simulink model "stepchange_timevarying_change"  (R2022b)
settings: Solver=VariableStepAuto  StartTime=0.0  StopTime=8  RelTol=1e-3
values from neighbouring files (symbols this model uses):
  A = [eye(N),     -LoadZ^-1,   B; zeros(BN,N),  R_l^-1*B',   eye(BN); zeros(1,N),  zeros(1,N),   V_r'*B ]    [stepchange_timevarying_change_initial_document.m]
  A_r = kron(diag(r),eye(N+BN+1))    [stepchange_timevarying_change_initial_document.m]
  alpha_u = [1.1    1.4    1.8    1.1           1.1    1.9    1.9    1.2           1.3    1.4    1.8    0.6           1.8    2.1    1.5    0.9]'    [stepchange_timevarying_change_initial_document.m]
  alpha_V = [0.7    0.6    0.8    0.9           0.7    1.2    0.8    1.24           0.3    0.3    0.0    1.70           1.0    0.5    1.1    1.0]'    [stepchange_timevarying_change_initial_document.m]
  alpha_w = 0.8    [stepchange_timevarying_change_initial_document.m]
  BN = size(Line1,1)/2    [stepchange_timevarying_change_initial_document.m]
  bound_up_vector = zeros(3*N,1)    [stepchange_timevarying_change_initial_document.m]
  changerate = 3    [stepchange_timevarying_change_initial_document.m]
  changetime = 5    [stepchange_timevarying_change_initial_document.m]
  changevariance = 0.1    [stepchange_timevarying_change_initial_document.m]
  constraint_gain = 200    [stepchange_timevarying_change_initial_document.m]
  Dw = 0.01    [stepchange_timevarying_change_initial_document.m]
  epsilon = 2    [stepchange_timevarying_change_initial_document.m]
  F_x = blkdiag(diag(r)*diag(alpha_I)+diag(r)*pr*diag(V_r),diag(r)*diag(alpha_V),F_x_I)    [stepchange_timevarying_change_initial_document.m]
  kappa = 10    [stepchange_timevarying_change_initial_document.m]
  l = 2.5    [stepchange_timevarying_change_initial_document.m]
  lambda_ini = zeros(N*(BN+N+1),1)    [stepchange_timevarying_change_initial_document.m]
  Lap = 1000*(Degree-Adjacent)    [stepchange_timevarying_change_initial_document.m]
  Lap_BN_plus_N = kron(Lap,eye(BN+N+1))    [stepchange_timevarying_change_initial_document.m]
  Lineconstrants = 10*ones(BN,1)    [stepchange_timevarying_change_initial_document.m]
  Lineindex = zeros(BN,4)    [stepchange_timevarying_change_initial_document.m]
  LoadI = [30.0;15.0;30.0;26.0;         18.9;22.8;29.6;32.1;         22.6;27.6;16.5;19.9;         26.5;19.4;22.7;24.9]    [stepchange_timevarying_change_initial_document.m]
  LoadIchange = [30.0;15.0;30.0;26.0;         18.9;22.8;29.6;32.1;         22.6;27.6;16.5;19.9;         26.5;19.4;22.7;24.9]+3*ones(N,1)    [stepchange_timevarying_change_initial_document.m]
  LoadIchangeno = 3    [stepchange_timevarying_change_initial_document.m]
  LoadZ = diag([16.7;50.0;16.7;20.0;              25.0;16.0;14.2;29.4;              18.5;19.6;22.6;25.6;              23.4;26.4;25.2;33.7])    [stepchange_timevarying_change_initial_document.m]
  LoadZchange = diag([16.7;50.0;16.7;20.0;              25.0;16.0;14.2;29.4;              18.5;19.6;22.6;25.6;              23.4;26.4;25.2;33.7])+3*diag(ones(N,1))    [stepchange_timevarying_change_initial_document.m]
  LoadZchangeno = 3    [stepchange_timevarying_change_initial_document.m]
  N = 16    [stepchange_timevarying_change_initial_document.m]
  NCLN = zeros(N,1)    [stepchange_timevarying_change_initial_document.m]
  normal_vector = zeros(3*N,1)    [stepchange_timevarying_change_initial_document.m]
  nu_ini = [-0.00758212493845042	-0.0182492317603708	0.00714905390846842	0.0186908981861182          -0.00758212493845042	-0.0182492317603708	0.00714905390846842	0.0186908981861182          -0.00758212493845042	-0.0182492317603708	0.00714905390846842	0.0186908981861182          -0.00758212493845042	-0.0182492317603708	0.00714905390846842	0.0186908981861182]'    [stepchange_timevarying_change_initial_document.m]
  pr = 0.005    [stepchange_timevarying_change_initial_document.m]
  r = [1.06 1.03 1.05 1.04     1.02 1.03 1.04 1.01     1.03 1.04 1.06 1.07     1.01 1.03 1.04 1.02]    [stepchange_timevarying_change_initial_document.m]
  s_A = zeros(N*(N+BN+1),1)    [stepchange_timevarying_change_initial_document.m]
  theta_ini = zeros(N*(BN+N+1),1)    [stepchange_timevarying_change_initial_document.m]
  u_ini = [378.9289  380.4146  379.7396  379.2243  380.1955  381.1042         379.9247  379.8974  380.0252  380.4045  379.6763  379.8341         380.1194  380.5682  379.3881  379.9696]'    [stepchange_timevarying_change_initial_document.m]
  upsilon_ini = [172.552238898892	172.552238898892	172.552238898892	172.552238898892               172.552238898892	172.552238898892	172.552238898892	172.552238898892               172.552238898892	172.552238898892	172.552238898892	172.552238898892               172.552238898892	172.552238898892	172.552238898892	172.552238898892]'    [stepchange_timevarying_change_initial_document.m]
  V_hat_low = (380-3)*ones(N,1)    [stepchange_timevarying_change_initial_document.m]
  V_hat_up = (380+3)*ones(N,1)    [stepchange_timevarying_change_initial_document.m]
  V_r = [380.16  381.31  380.27  380.13       380.12  381.24  380.15  380.35       380.15  381.13  380.09  380.22       380.19  381.26  380.21  380.19]'    [stepchange_timevarying_change_initial_document.m]
  varepsilon = 50    [stepchange_timevarying_change_initial_document.m]
  x_hat_ini = [14.515064754915	3.95935897697232	32.9787419273847	14.9071228299889             37.6257931691129	61.1095883901259	41.4721611959256	33.6364102939300             44.9867290171943	52.8132621486412	28.1355733315040	33.0707668633162             36.6024320622732	49.3936276267038	2.38033527987224	36.4476162672594             378.638597580330	380.343321138855	379.211948658584	379.000752058610              ...(+639 chars)    [stepchange_timevarying_change_initial_document.m]
undefined symbols (not defined in the file or in its folder): bound_low_vector
libraries: fl_lib x204, nesl_utility x101, simulink x2, spspowerguiLib x1
(part 1 of 3)
settings Model: Creator=27843  LastModifiedBy=27843

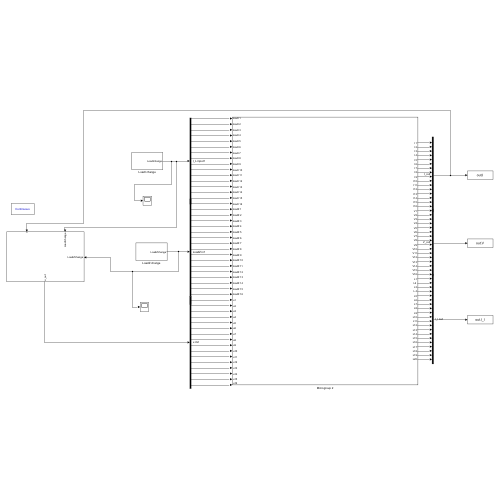
[thumbnail: Simulink's stored preview of the top-level diagram]
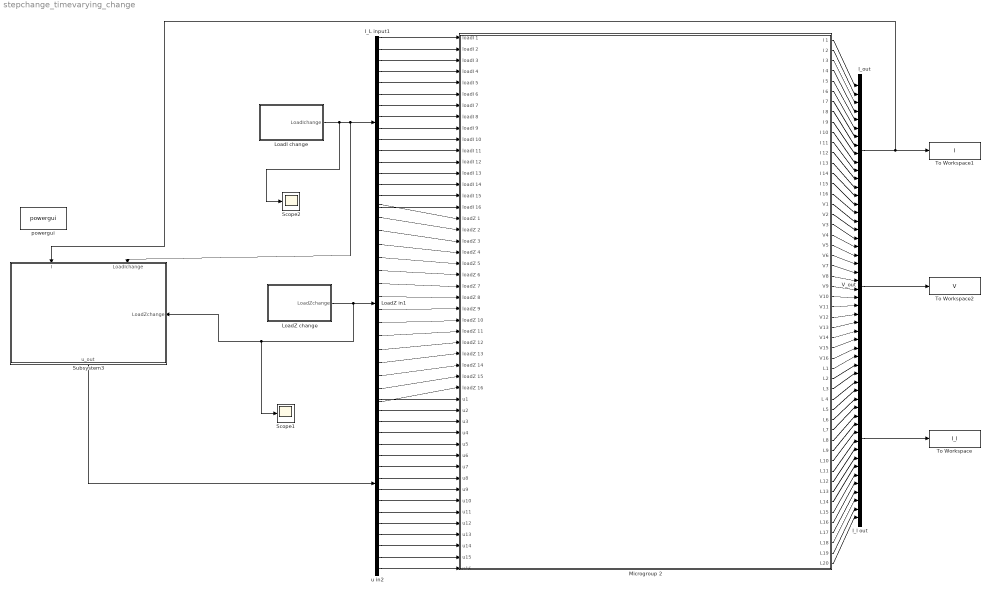
== system stepchange_timevarying_change ==
  I_L input1 : Demux  Outputs=16
  I_l out : Mux  Inputs=20
  I_out : Mux  Inputs=16
  LoadI change : Subsystem
  LoadZ change : Subsystem
  LoadZ in1 : Demux  Outputs=16
  Microgroup 2 : Subsystem
  Scope1 : Scope
  Scope2 : Scope
  Subsystem3 : Subsystem
      settings: PortSchema="{\"entries\":[{\"content\":{\"sides\":[{\"content\":{\"connectorIds\":[\"In1\",\"In2\"]},\"type\":\"ConnectorPlacement.EquallySpacedRectSide\",\"uuid\":\"fae7fbbb-70cd-4db5-acb5-97da1dd1ec52\"},{\"content\":{\"connectorIds\":[\"Out1\"],\"side\":\"RIGHT\"},\"type\":\"ConnectorPlacement.EquallySpacedRectSide\",\"uuid\":\"fa6dcfc8-22a3-4b8e-9bd6-bb4867dcf5b7\"},{\"content\":{\"connectorIds\":[],\"side\":\"TOP\"},\"type\":\"ConnectorPlacement.EquallySpacedRectSide\",\"uuid\":\"9780a6fc-e699-499b-ab3e-b386f79a2eae\"},{\"content\":{\"connectorIds\":[\"In3\"],\"side\":\"BOTTOM\"},\"type\":\"ConnectorPlacement.EquallySpacedRectSide\",\"uuid\":\"c19162d8-377f-47b4-a15d-68590b7e29f2\"}]},\"type\":\"ConnectorPlacement.EquallySpacedConnector\",\"uuid\":\"94524866-4569-4101-9a5a-19d024da94d3\"}],\"packageUris\":[\"http://schema.mathworks.com/mf0/Connector/R2020b\"],\"version\":\"1.0\"}"
  To Workspace : ToWorkspace  VariableName=I_l  SaveFormat=Timeseries  SampleTime=-1
  To Workspace1 : ToWorkspace  VariableName=I  SaveFormat=Timeseries  SampleTime=-1
  To Workspace2 : ToWorkspace  VariableName=V  SaveFormat=Timeseries  SampleTime=-1
  V_out : Mux  Inputs=16
  powergui : spspowerguiLib/powergui  Priority=1  SimulationMode=Continuous  SampleTime=50e-6  frequency=60  Iterations=50  frequencyindice=60  Pbase=100e6  ErrMax=1e-4  UnitsV=kV  UnitsW=MW  buscounter=0  FunctionMessages=off  echomessages=off  EnableUseOfTLC=off  CurrentSourceSwitches=off  DisableSnubberDevices=off  DisableRonSwitches=off  DisableVfSwitches=off  DisplayEquations=off  AutomaticDiscreteSolvers=off  SolverType=Tustin/Backward Euler (TBE)  Interpol=off  ExternalGateDelay=off  methode=off  Ts=100  x0status=blocks  SPID=on  SwTol=0  HookPort=off  NonlinearTolerance=1e-4  nMaxIteration=100  ContinueOnMaxIteration=off  RestoreLinks=warning  ResistiveCurrentMeasurement=off  Frange=[0:2:500]  Ylog=off  Xlog=on  ShowGrid=off  save=off  variable=ZData  structure=0  ZoomFFT=off  StartTime=0.0  cycles=1  DisplayStyle=1  fundamental=60  FreqAxis=off  MaxFrequency=1000  frequencyindicesteady=1  RmsSteady=1  display=off
  u in2 : Demux  Outputs=16
  wires:
  Microgroup 2/25(V9) -> V_out/9
  Microgroup 2/11(I 11) -> I_out/11
  I_L input1/14 -> Microgroup 2/14(loadI 14)
  LoadI change/1(LoadIchange) -> Scope2/1, I_L input1/1, Subsystem3/2(LoadIchange)
  Microgroup 2/23(V7) -> V_out/7
  LoadZ change/1(LoadZchange) -> Scope1/1, Subsystem3/3(LoadZchange), LoadZ in1/1
  Microgroup 2/20(V4) -> V_out/4
  V_out/1 -> To Workspace2/1
  Microgroup 2/8(I 8) -> I_out/8
  Microgroup 2/27(V11) -> V_out/11
  LoadZ in1/3 -> Microgroup 2/19(loadZ 3)
  I_L input1/10 -> Microgroup 2/10(loadI 10)
  u in2/13 -> Microgroup 2/45(u13)
  LoadZ in1/10 -> Microgroup 2/26(loadZ 10)
  u in2/11 -> Microgroup 2/43(u11)
  I_L input1/5 -> Microgroup 2/5(loadI 5)
  I_L input1/8 -> Microgroup 2/8(loadI 8)
  Subsystem3/1(u_out) -> u in2/1
  I_L input1/16 -> Microgroup 2/16(loadI 16)
  u in2/15 -> Microgroup 2/47(u15)
  LoadZ in1/11 -> Microgroup 2/27(loadZ 11)
  I_l out/1 -> To Workspace/1
  LoadZ in1/9 -> Microgroup 2/25(loadZ 9)
  I_out/1 -> To Workspace1/1, Subsystem3/1(I)
  u in2/12 -> Microgroup 2/44(u12)
  Microgroup 2/15(I 15) -> I_out/15
  LoadZ in1/5 -> Microgroup 2/21(loadZ 5)
  u in2/4 -> Microgroup 2/36(u4)
  Microgroup 2/6(I 6) -> I_out/6
  u in2/5 -> Microgroup 2/37(u5)
  u in2/7 -> Microgroup 2/39(u7)
  u in2/8 -> Microgroup 2/40(u8)
  u in2/2 -> Microgroup 2/34(u2)
  LoadZ in1/6 -> Microgroup 2/22(loadZ 6)
  Microgroup 2/51(L19) -> I_l out/19
  I_L input1/3 -> Microgroup 2/3(loadI 3)
  Microgroup 2/39(" L7") -> I_l out/7
  u in2/3 -> Microgroup 2/35(u3)
  u in2/1 -> Microgroup 2/33(u1)
  LoadZ in1/4 -> Microgroup 2/20(loadZ 4)
  Microgroup 2/48(L16) -> I_l out/16
  Microgroup 2/42(L10) -> I_l out/10
  Microgroup 2/41(L9) -> I_l out/9
  Microgroup 2/46(L14) -> I_l out/14
  Microgroup 2/36(L 4) -> I_l out/4
  Microgroup 2/44(L12) -> I_l out/12
  Microgroup 2/38(L6) -> I_l out/6
  Microgroup 2/16(I 16) -> I_out/16
  Microgroup 2/47(L15) -> I_l out/15
  Microgroup 2/14(I 14) -> I_out/14
  Microgroup 2/13(I 13) -> I_out/13
  u in2/10 -> Microgroup 2/42(u10)
  Microgroup 2/22(V6) -> V_out/6
  Microgroup 2/49(L17) -> I_l out/17
  Microgroup 2/33(L1) -> I_l out/1
  Microgroup 2/52(L20) -> I_l out/20
  u in2/14 -> Microgroup 2/46(u14)
  Microgroup 2/18(V2) -> V_out/2
  Microgroup 2/26(V10) -> V_out/10
  u in2/6 -> Microgroup 2/38(u6)
  Microgroup 2/17(V1) -> V_out/1
  Microgroup 2/21(V5) -> V_out/5
  Microgroup 2/50(L18) -> I_l out/18
  Microgroup 2/29(V13) -> V_out/13
  Microgroup 2/19(V3) -> V_out/3
  Microgroup 2/2(I 2) -> I_out/2
  Microgroup 2/43(" L11") -> I_l out/11
  Microgroup 2/7(I 7) -> I_out/7
  LoadZ in1/1 -> Microgroup 2/17(loadZ 1)
  Microgroup 2/5(I 5) -> I_out/5
  Microgroup 2/40(L8) -> I_l out/8
  LoadZ in1/16 -> Microgroup 2/32(loadZ 16)
  I_L input1/1 -> Microgroup 2/1(loadI 1)
  Microgroup 2/35(L3) -> I_l out/3
  Microgroup 2/31(V15) -> V_out/15
  Microgroup 2/1(I 1) -> I_out/1
  LoadZ in1/14 -> Microgroup 2/30(loadZ 14)
  LoadZ in1/7 -> Microgroup 2/23(loadZ 7)
  u in2/9 -> Microgroup 2/41(u9)
  Microgroup 2/4(I 4) -> I_out/4
  LoadZ in1/8 -> Microgroup 2/24(loadZ 8)
  Microgroup 2/34("L2 ") -> I_l out/2
  Microgroup 2/37(L5) -> I_l out/5
  I_L input1/6 -> Microgroup 2/6(loadI 6)
  Microgroup 2/30(V14) -> V_out/14
  I_L input1/2 -> Microgroup 2/2(loadI 2)
  LoadZ in1/12 -> Microgroup 2/28(loadZ 12)
  Microgroup 2/9(I 9) -> I_out/9
  Microgroup 2/3(I 3) -> I_out/3
  Microgroup 2/12(I 12) -> I_out/12
  I_L input1/9 -> Microgroup 2/9(loadI 9)
  LoadZ in1/13 -> Microgroup 2/29(loadZ 13)
  Microgroup 2/45(L13) -> I_l out/13
  I_L input1/13 -> Microgroup 2/13(loadI 13)
  Microgroup 2/24(V8) -> V_out/8
  LoadZ in1/2 -> Microgroup 2/18(loadZ 2)
  Microgroup 2/28(V12) -> V_out/12
  Microgroup 2/10(I 10) -> I_out/10
  Microgroup 2/32(V16) -> V_out/16
  I_L input1/11 -> Microgroup 2/11(loadI 11)
  I_L input1/4 -> Microgroup 2/4(loadI 4)
  I_L input1/15 -> Microgroup 2/15(loadI 15)
  I_L input1/12 -> Microgroup 2/12(loadI 12)
  u in2/16 -> Microgroup 2/48(u16)
  I_L input1/7 -> Microgroup 2/7(loadI 7)
  LoadZ in1/15 -> Microgroup 2/31(loadZ 15)

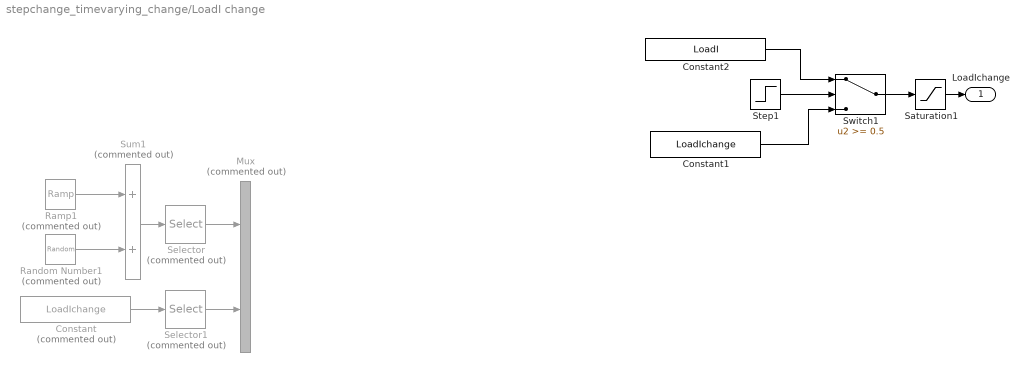
== system stepchange_timevarying_change/LoadI change ==
  Constant : Constant  Commented=on  Value=LoadIchange
  Constant1 : Constant  Value=LoadIchange
  Constant2 : Constant  Value=LoadI
  Mux : Mux  Commented=on  Inputs=2
  Ramp1 : simulink/Sources/Ramp  Commented=on  slope=changerate  start=changetime  InitialOutput=LoadIchange
  Random Number1 : RandomNumber  Commented=on  Variance=changevariance  SampleTime=0.01
  Saturation1 : Saturate  UpperLimit=LoadI+LoadIchangeno*ones(N,1)
  Selector : Selector  Commented=on  InputPortWidth=16  IndexOptions=Index vector (dialog)  Indices=[1:8]  OutputSizes=1
  Selector1 : Selector  Commented=on  InputPortWidth=16  IndexOptions=Index vector (dialog)  Indices=[9:16]  OutputSizes=1
  Step1 : Step  Time=changetime  Before=1  After=0  SampleTime=0
  Sum1 : Sum  Commented=on
  Switch1 : Switch  Threshold=0.5  SaturateOnIntegerOverflow=off  InputSameDT=off
  LoadIchange : Outport
  wires:
  Step1/1 -> Switch1/2
  Switch1/1 -> Saturation1/1
  Constant2/1 -> Switch1/1
  Saturation1/1 -> LoadIchange/1
  Selector/1 -> Mux/1
  Random Number1/1 -> Sum1/2
  Selector1/1 -> Mux/2
  Ramp1/1 -> Sum1/1
  Constant/1 -> Selector1/1
  Sum1/1 -> Selector/1
  Constant1/1 -> Switch1/3

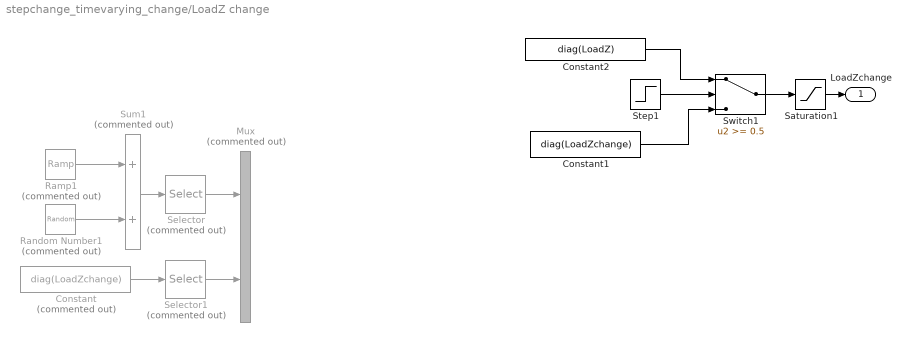
== system stepchange_timevarying_change/LoadZ change ==
  Constant : Constant  Commented=on  Value=diag(LoadZchange)
  Constant1 : Constant  Value=diag(LoadZchange)
  Constant2 : Constant  Value=diag(LoadZ)
  Mux : Mux  Commented=on  Inputs=2
  Ramp1 : simulink/Sources/Ramp  Commented=on  slope=changerate  start=changetime  InitialOutput=diag(LoadZ)
  Random Number1 : RandomNumber  Commented=on  Variance=changevariance  SampleTime=0.01
  Saturation1 : Saturate  UpperLimit=diag(LoadZ)+LoadZchangeno*ones(N,1)
  Selector : Selector  Commented=on  InputPortWidth=16  IndexOptions=Index vector (dialog)  Indices=[1:8]  OutputSizes=1
  Selector1 : Selector  Commented=on  InputPortWidth=16  IndexOptions=Index vector (dialog)  Indices=[9:16]  OutputSizes=1
  Step1 : Step  Time=changetime  Before=1  After=0  SampleTime=0
  Sum1 : Sum  Commented=on
  Switch1 : Switch  Threshold=0.5  SaturateOnIntegerOverflow=off  InputSameDT=off
  LoadZchange : Outport
  wires:
  Switch1/1 -> Saturation1/1
  Ramp1/1 -> Sum1/1
  Step1/1 -> Switch1/2
  Constant2/1 -> Switch1/1
  Random Number1/1 -> Sum1/2
  Saturation1/1 -> LoadZchange/1
  Sum1/1 -> Selector/1
  Selector/1 -> Mux/1
  Constant/1 -> Selector1/1
  Selector1/1 -> Mux/2
  Constant1/1 -> Switch1/3
